simulink model "P3redosim"  (R2022a)
settings: Solver=VariableStepAuto  StartTime=ts  StopTime=tf  FixedStep=tstep  RelTol=1e-3
settings Model: Creator=nsm0014  LastModifiedBy=nsm0014

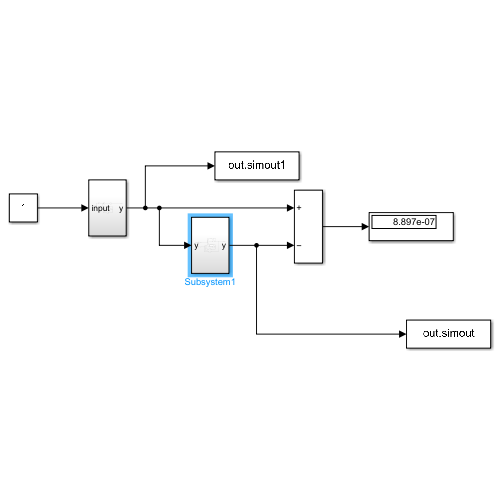
[thumbnail: Simulink's stored preview of the top-level diagram]
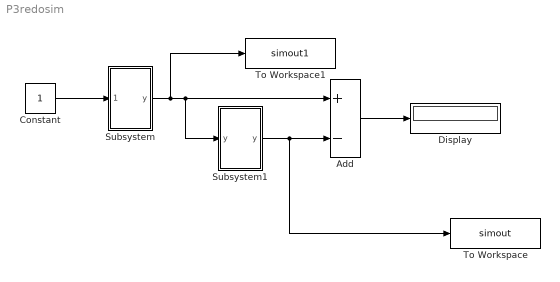
== system P3redosim ==
  Add : Sum  Inputs=+-
  Constant : Constant
  Display : Display
  Subsystem : Subsystem
  Subsystem1 : Subsystem
  To Workspace : ToWorkspace  VariableName=simout  SaveFormat=Structure With Time  SampleTime=-1
  To Workspace1 : ToWorkspace  VariableName=simout1  SaveFormat=Structure With Time  SampleTime=-1
  wires:
  Subsystem/1(y) -> To Workspace1/1, Subsystem1/1("y "), Add/1
  Subsystem1/1(y) -> To Workspace/1, Add/2
  Add/1 -> Display/1
  Constant/1 -> Subsystem/1(input)

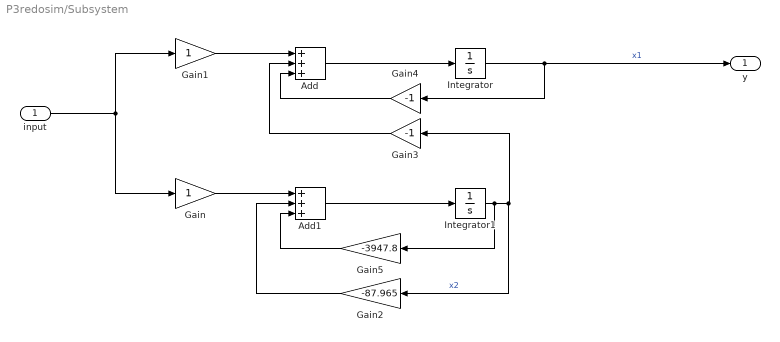
== system P3redosim/Subsystem ==
  input : Inport
  Add : Sum  Inputs=+++
  Add1 : Sum  Inputs=+++
  Gain : Gain
  Gain1 : Gain
  Gain2 : Gain  Gain=-87.965
  Gain3 : Gain  Gain=-1
  Gain4 : Gain  Gain=-1
  Gain5 : Gain  Gain=-3947.8
  Integrator : Integrator
  Integrator1 : Integrator
  y : Outport
  wires:
  Gain1/1 -> Add/1
  Integrator/1 -> Gain4/1, y/1  "x1"
  Integrator1/1 -> Gain5/1, Gain3/1, Gain2/1  "x2"
  Gain/1 -> Add1/1
  Gain2/1 -> Add1/2
  input/1 -> Gain/1, Gain1/1
  Add1/1 -> Integrator1/1
  Add/1 -> Integrator/1
  Gain3/1 -> Add/2
  Gain4/1 -> Add/3
  Gain5/1 -> Add1/3

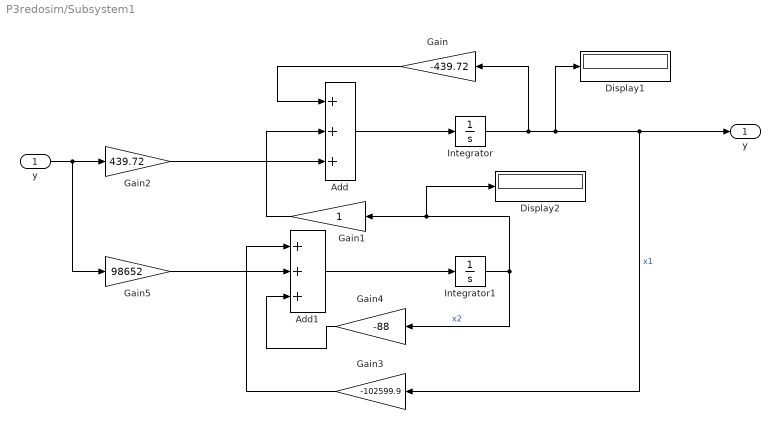
== system P3redosim/Subsystem1 ==
  "y " : Inport
  Add : Sum  Inputs=+++
  Add1 : Sum  Inputs=+++
  Display1 : Display
  Display2 : Display
  Gain : Gain  Gain=-439.72
  Gain1 : Gain
  Gain2 : Gain  Gain=439.72
  Gain3 : Gain  Gain=-102599.9
  Gain4 : Gain  Gain=-88
  Gain5 : Gain  Gain=98652
  Integrator : Integrator
  Integrator1 : Integrator
  y : Outport
  wires:
  Integrator1/1 -> Display2/1, Gain1/1, Gain4/1  "x2"
  Integrator/1 -> Gain/1, Display1/1, Gain3/1, y/1  "x1"
  Add/1 -> Integrator/1
  Gain/1 -> Add/1
  Gain2/1 -> Add/3
  "y "/1 -> Gain5/1, Gain2/1
  Gain5/1 -> Add1/2
  Gain4/1 -> Add1/3
  Gain3/1 -> Add1/1
  Add1/1 -> Integrator1/1
  Gain1/1 -> Add/2
